simulink model "signalbuilder"  (R2022b)
settings: Solver=VariableStepAuto  StartTime=0.0  StopTime=10.0  RelTol=1e-3
undefined symbols (not defined in the file): sigbuilder_block
settings Model: Creator=Brigosha_guest  LastModifiedBy=Brigosha_guest

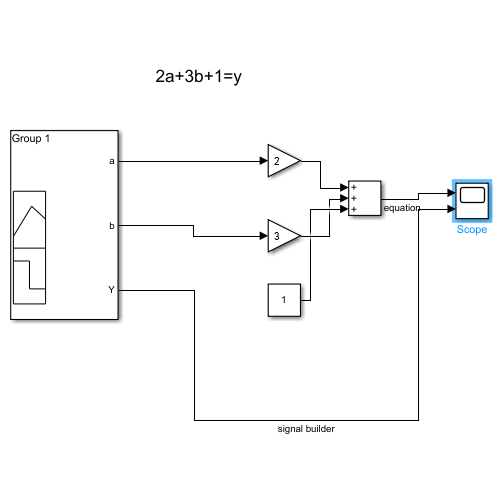
[thumbnail: Simulink's stored preview of the top-level diagram]
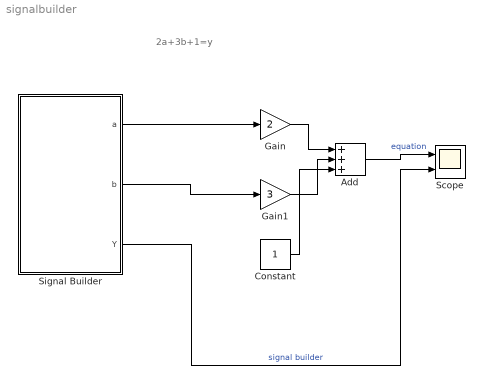
== system signalbuilder ==
  note: 2a+3b+1=y
  Add : Sum  Inputs=+++
  Constant : Constant
  Gain : Gain  Gain=2
  Gain1 : Gain  Gain=3
  Scope : Scope  NumInputPorts=2
  Signal Builder : Subsystem  Tag=STV Subsys  LoadFcn=sigbuilder_block('load');  StartFcn=sigbuilder_block('start');  StopFcn=sigbuilder_block('stop');  ClipboardFcn=sigbuilder_block('clipboard');  mask(Sigbuilder block){tuvar=[0:10]}
      mask help: Simulink:masks:SigbuilderBlock_MD
      mask init:
      | if ~strcmp(get_param(bdroot(gcbh),'SimulationStatus'),'stopped') tuvar = sigbuilder_block('maskInit'); end
      settings: CopyFcn=sigbuilder_block('copy');  DeleteFcn=sigbuilder_block('delete');  ModelCloseFcn=sigbuilder_block('modelClose');  PreSaveFcn=sigbuilder_block('preSave');  PauseFcn=sigbuilder_block('pause');  ContinueFcn=sigbuilder_block('continue');  NameChangeFcn=sigbuilder_block('namechange');  OpenFcn=sigbuilder_block('open',[369.75 22.5 550.5 359.25 ]);  CloseFcn=sigbuilder_block('close');
      mask Display: plot(0, 0, 100, 100,[2, 2, 32, 32, 2], [68, 8, 8, 68, 68],[32, 2], [38, 38], [32, 19, 2],[53, 60, 44], [32, 17, 17, 2],[16, 16, 31, 31]);txt = getActiveGroup(gcbh);text(2, 100, txt,'verticalAlignment', 'top');
  wires:
  Gain/1 -> Add/1
  Gain1/1 -> Add/2
  Constant/1 -> Add/3
  Add/1 -> Scope/1  "equation"
  Signal Builder/1(a) -> Gain/1
  Signal Builder/2(b) -> Gain1/1
  Signal Builder/3(Y) -> Scope/2  "signal builder"

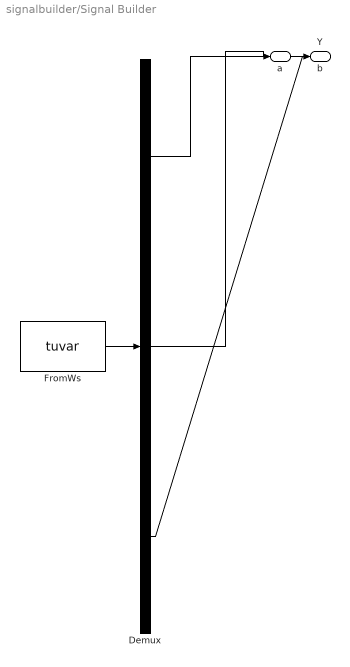
== system signalbuilder/Signal Builder ==
  Demux : Demux  Tag=STV Demux  Outputs=3
      settings: DisplayOption=none
  FromWs : FromWorkspace  Tag=STV FromWs  VariableName=tuvar
      SigBuilderData=|
      | common.afterFinalStr = 'Extrapolate'
      | common.sampleTime = 0
      | dataSet.timeRange = [0 10]
      | dataSet.name = 'Group 1'
      | sbobj.Groups.Name = 'Group 1'
      | sbobj.Groups.Signals(1).Name = 'a'
      | sbobj.Groups.Signals(1).XData = [0 3 3 7.96 7.96 10]
      | sbobj.Groups.Signals(1).YData = [0.04 0.04 2 2 0 0]
      | sbobj.Groups.Signals(2).Name = 'b'
      | sbobj.Groups.Signals(2).XData = [0 4 4 9 9 10]
      | sbobj.Groups.Signals(2).YData = [0 0 3 3 0 0]
      | sbobj.Groups.Signals(3).Name = 'Y'
      | sbobj.Groups.Signals(3).XData = [0 1 1 2 3 3 4 4 5 6 7 8 8 9 9 10]
      | sbobj.Groups.Signals(3).YData = [1 1 1.05 1.05 1.05 5 5 14 14 14 14 14 10 10 1 1]
  a : Outport  Tag=STV Outport
  b : Outport  Tag=STV Outport  Port=2
  Y : Outport  Tag=STV Outport  Port=3
  wires:
  Demux/1 -> a/1
  FromWs/1 -> Demux/1
  Demux/2 -> b/1
  Demux/3 -> Y/1
